simulink model "SIMMODEL"  (R2023b)
settings: Solver=VariableStepAuto  StartTime=0.0  StopTime=1.2  MaxStep=0.2  RelTol=1e-4  EnableMultiTasking=on
libraries: spsThreePhaseFaultLib x12, spsDistributedParametersLineLib x2, spsMutualInductanceLib x2, spsThreePhaseSourceLib x2, spsThreePhaseVIMeasurementLib x1, spspowerguiLib x1
settings Model: Creator=t0197si  LastModifiedBy=takid
settings SolverCC: AlgebraicLoopSolver=TrustRegion  MaxZcPerStep=1
settings DataIOCC: LimitDataPoints=on  MaxDataPoints=10000
settings OptimizationCC: ReuseModelBlockBuffer=off  LifeSpan=inf
settings DebuggingCC: UnconnectedInputMsg=warning  UnconnectedOutputMsg=warning  UnconnectedLineMsg=warning  AllowSymbolicDim=off  SFUnexpectedBacktrackingDiag=warning  SFNoUnconditionalDefaultTransitionDiag=warning  SFExecutionAtInitializationDiag=none  ArithmeticOperatorsInVariantConditions=warning
settings ModelReferenceCC: EnableRefExpFcnMdlSchedulingChecks=on
settings SFSimCC: SimUseLocalCustomCode=off  CustomCodeUndefinedFunction=UseInterfaceOnly
settings RTWCC: RTWUseLocalCustomCode=off  DLArmComputeVersion=19.05
settings CodeAppCC: StateflowObjectComments=on
settings GRTTargetCC: TargetLangStandard=C89/C90 (ANSI)
settings ConfigComp: CovMetricSettings=dw  CovSaveCumulativeToWorkspaceVar=on  CovSaveSingleToWorkspaceVar=on  CovExternalEMLEnable=off  CovSFcnEnable=off
settings SimscapeCC: SimscapeLogType=all  SimscapeLogDataHistory=10000

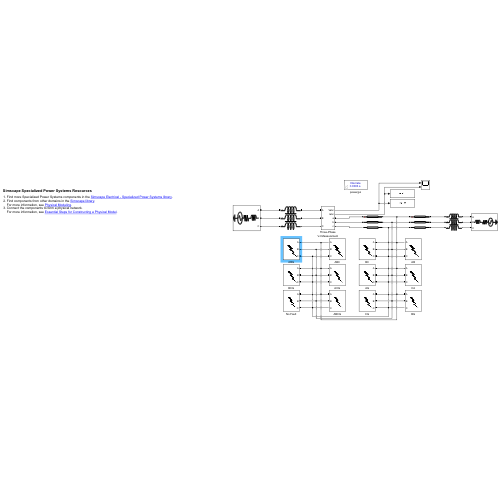
[thumbnail: Simulink's stored preview of the top-level diagram]
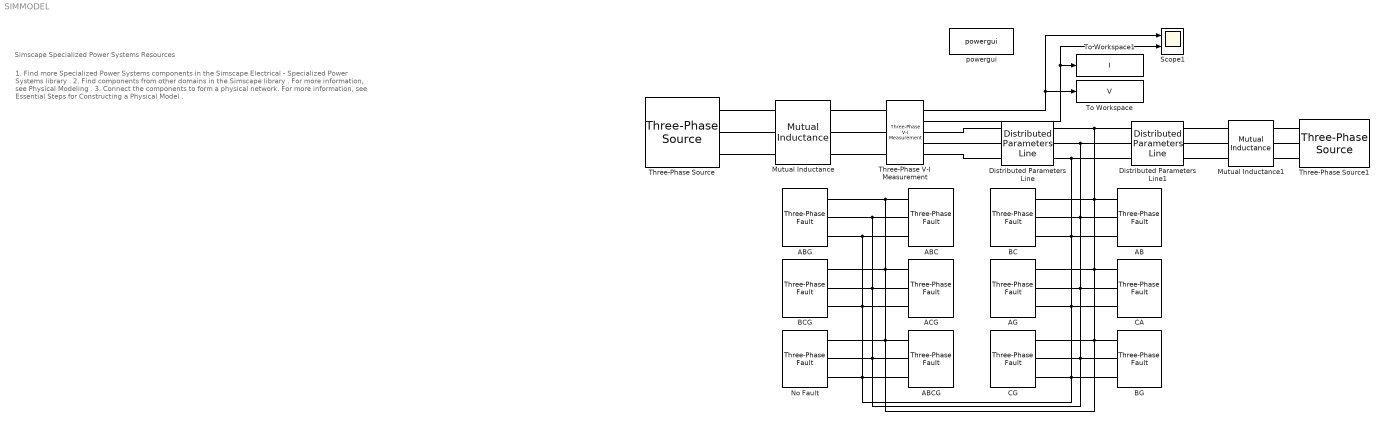
== system SIMMODEL ==
  note: 1. Find more Specialized Power Systems components in the Simscape Electrical - Specialized Power Systems library .
      | 2. Find components from other domains in the Simscape library .
      | For more information, see Physical Modeling .
      | 3. Connect the components to form a physical network.
      | For more information, see Essential Steps for Constructing a Physical Model .
  note: Simscape Specialized Power Systems Resources
  AB : spsThreePhaseFaultLib/Three-Phase Fault  InitialStates=0  FaultA=on  FaultB=on  FaultC=off  GroundFault=off  SwitchTimes="[0.048  0.051]"  External=off  SwitchStatus=NaN  FaultResistance=0.0001  GroundResistance=0.01  SnubberResistance=1e6  SnubberCapacitance=inf  Measurements=Fault voltages and currents
  ABC : spsThreePhaseFaultLib/Three-Phase Fault  InitialStates=0  FaultA=on  FaultB=on  FaultC=on  GroundFault=off  SwitchTimes="[0.648  0.651]"  External=off  SwitchStatus=NaN  FaultResistance=0.0001  GroundResistance=0.01  SnubberResistance=1e6  SnubberCapacitance=inf  Measurements=Fault voltages and currents
  ABCG : spsThreePhaseFaultLib/Three-Phase Fault  InitialStates=0  FaultA=on  FaultB=on  FaultC=on  GroundFault=on  SwitchTimes="[1.05  1.053]"  External=off  SwitchStatus=NaN  FaultResistance=0.0001  GroundResistance=0.01  SnubberResistance=1e6  SnubberCapacitance=inf  Measurements=Fault voltages and currents
  ABG : spsThreePhaseFaultLib/Three-Phase Fault  InitialStates=0  FaultA=on  FaultB=on  FaultC=off  GroundFault=on  SwitchTimes="[0.75  0.753]"  External=off  SwitchStatus=NaN  FaultResistance=0.0001  GroundResistance=0.01  SnubberResistance=1e6  SnubberCapacitance=inf  Measurements=Fault voltages and currents
  ACG : spsThreePhaseFaultLib/Three-Phase Fault  InitialStates=0  FaultA=on  FaultB=off  FaultC=on  GroundFault=on  SwitchTimes="[0.849  0.852]"  External=off  SwitchStatus=NaN  FaultResistance=0.0001  GroundResistance=0.01  SnubberResistance=1e6  SnubberCapacitance=inf  Measurements=Fault voltages and currents
  AG : spsThreePhaseFaultLib/Three-Phase Fault  InitialStates=0  FaultA=on  FaultB=off  FaultC=off  GroundFault=on  SwitchTimes="[0.348  0.351]"  External=off  SwitchStatus=NaN  FaultResistance=0.0001  GroundResistance=0.01  SnubberResistance=1e6  SnubberCapacitance=inf  Measurements=Fault voltages and currents
  BC : spsThreePhaseFaultLib/Three-Phase Fault  InitialStates=0  FaultA=off  FaultB=on  FaultC=on  GroundFault=off  SwitchTimes="[0.150  0.153]"  External=off  SwitchStatus=NaN  FaultResistance=0.0001  GroundResistance=0.01  SnubberResistance=1e6  SnubberCapacitance=inf  Measurements=Fault voltages and currents
  BCG : spsThreePhaseFaultLib/Three-Phase Fault  InitialStates=0  FaultA=off  FaultB=on  FaultC=on  GroundFault=on  SwitchTimes="[0.948  0.951]"  External=off  SwitchStatus=NaN  FaultResistance=0.0001  GroundResistance=0.01  SnubberResistance=1e6  SnubberCapacitance=inf  Measurements=Fault voltages and currents
  BG : spsThreePhaseFaultLib/Three-Phase Fault  InitialStates=0  FaultA=off  FaultB=on  FaultC=off  GroundFault=on  SwitchTimes="[0.45  0.453]"  External=off  SwitchStatus=NaN  FaultResistance=0.0001  GroundResistance=0.01  SnubberResistance=1e6  SnubberCapacitance=inf  Measurements=Fault voltages and currents
  CA : spsThreePhaseFaultLib/Three-Phase Fault  InitialStates=0  FaultA=on  FaultB=off  FaultC=on  GroundFault=off  SwitchTimes="[0.249  0.252]"  External=off  SwitchStatus=NaN  FaultResistance=0.0001  GroundResistance=0.01  SnubberResistance=1e6  SnubberCapacitance=inf  Measurements=Fault voltages and currents
  CG : spsThreePhaseFaultLib/Three-Phase Fault  InitialStates=0  FaultA=off  FaultB=off  FaultC=on  GroundFault=on  SwitchTimes="[0.549  0.552]"  External=off  SwitchStatus=NaN  FaultResistance=0.0001  GroundResistance=0.01  SnubberResistance=1e6  SnubberCapacitance=inf  Measurements=Fault voltages and currents
  Distributed Parameters Line : spsDistributedParametersLineLib/Distributed Parameters Line  Phases=3  Length=100  Frequency=60  Resistance=[0.01273 0.3864]  Inductance="[0.9337e-3  4.1264e-3]"  Capacitance=[12.74e-9 7.751e-9]  x1=[-0.0006 8.38191360726551e-10 366849.409185142 -341970.613327489;-0.0003 9.78318632999942e-10 403099.289377047 -298384.57115405]  x2=[-0.0006 2.49160898759062e-08 369790.162967538 -345071.374185274;-0.0003 2.69712684545462e-08 406371.196257459 -301133.639372877]  x3=[-0.0006 -7.11140025193407e-11 1183.26211569335 -1433.40164787206;-0.0003 -5.12740809092146e-11 1337.47114951323 -1290.70540510875]  x4=[-0.0006 1.02696315275821e-10 1363.36060464342 -1272.22615544696;-0.0003 8.61930580244731e-11 1498.22936173638 -1110.23434847254]  x5=0.000565541566995742  V1=[2.072e-10 5.015e+05 5.015e+05;377 377 377;0.5654 0.9167 -0.6541]  V2=[3.283e-10 5.058e+05 5.058e+05;377 377 377;2.705 0.9161 -0.6547]  I1=[2.823e-12 1859 1859;377 377 377;1.555 0.7863 -0.7845]  I2=[3.303e-12 1865 1865;377 377 377;-0.9037 0.9161 -0.6547]  nHarmo=1  Measurements=None  Decoupling=off  VsMag0=0  VrMag0=0  VsAngle0=0  VrAngle0=0  IsMag0=0  IrMag0=0  IsAngle0=0  IrAngle0=0
      settings: LibrarySourceBlock=sps_lib/Power Grid Elements/Distributed Parameters Line
  Distributed Parameters Line1 : spsDistributedParametersLineLib/Distributed Parameters Line  Phases=3  Length=100  Frequency=60  Resistance=[0.01273 0.3864]  Inductance="[0.9337e-3  4.1264e-3]"  Capacitance=[12.74e-9 7.751e-9]  x1=[-0.0006 2.48987725575321e-08 369790.162967538 -345071.374185274;-0.0003 2.69552313818675e-08 406371.196257459 -301133.639372877]  x2=[-0.0006 1.02377184379559e-09 366849.409185141 -341970.613327489;-0.0003 1.14493289747496e-09 403099.289377047 -298384.57115405]  x3=[-0.0006 1.04415855312855e-10 1363.36060464343 -1272.22615544696;-0.0003 8.82283474754132e-11 1498.22936173639 -1110.23434847254]  x4=[-0.0006 -7.33549795214247e-11 1183.26211569334 -1433.40164787206;-0.0003 -5.35717652018444e-11 1337.47114951323 -1290.70540510875]  x5=0.000565541566995742  V1=[3.185e-10 5.058e+05 5.058e+05;377 377 377;2.745 0.9161 -0.6547]  V2=[1.2e-10 5.015e+05 5.015e+05;377 377 377;-0.4582 0.9167 -0.6541]  I1=[2.458e-12 1865 1865;377 377 377;-1.648 0.9161 -0.6547]  I2=[3.271e-12 1859 1859;377 377 377;1.776 0.7863 -0.7845]  nHarmo=1  Measurements=None  Decoupling=off  VsMag0=0  VrMag0=0  VsAngle0=0  VrAngle0=0  IsMag0=0  IrMag0=0  IsAngle0=0  IrAngle0=0
      settings: LibrarySourceBlock=sps_lib/Power Grid Elements/Distributed Parameters Line
  Mutual Inductance : spsMutualInductanceLib/Mutual Inductance  LConnTagsString=a|b|c  RConnTagsString=A|B|C  TypeOfMutual=Two or three windings with equal mutual terms  NumberOfWindings=3  SelfImpedance1=[1.1 1.1e-03]  SelfImpedance2=[ 1.1 1.1e-03]  ThreeWindings=on  SelfImpedance3=[ 1.1 1.1e-03]  MutualImpedance=[1.0 1.0e-03]  InductanceMatrix="[1.0 0.9  0.9 ;  0.9 1.0  0.9;  0.9 0.9 1.0 ] * 1e-3"  ResistanceMatrix="[1.0 0.9  0.9 ;  0.9 1.0  0.9;  0.9 0.9 1.0 ]"  Measurements=None
      settings: LibrarySourceBlock=sps_lib/Passives/Mutual Inductance
  Mutual Inductance1 : spsMutualInductanceLib/Mutual Inductance  LConnTagsString=a|b|c  RConnTagsString=A|B|C  TypeOfMutual=Two or three windings with equal mutual terms  NumberOfWindings=3  SelfImpedance1=[1.1 1.1e-03]  SelfImpedance2=[ 1.1 1.1e-03]  ThreeWindings=on  SelfImpedance3=[ 1.1 1.1e-03]  MutualImpedance=[1.0 1.0e-03]  InductanceMatrix="[1.0 0.9  0.9 ;  0.9 1.0  0.9;  0.9 0.9 1.0 ] * 1e-3"  ResistanceMatrix="[1.0 0.9  0.9 ;  0.9 1.0  0.9;  0.9 0.9 1.0 ]"  Measurements=None
      settings: LibrarySourceBlock=sps_lib/Passives/Mutual Inductance
  No Fault : spsThreePhaseFaultLib/Three-Phase Fault  InitialStates=0  FaultA=off  FaultB=off  FaultC=off  GroundFault=off  SwitchTimes="[1.15  1.151]"  External=off  SwitchStatus=NaN  FaultResistance=0.0001  GroundResistance=0.01  SnubberResistance=1e6  SnubberCapacitance=inf  Measurements=Fault voltages and currents
  Scope1 : Scope  NumInputPorts=2
  Three-Phase V-I Measurement : spsThreePhaseVIMeasurementLib/Three-Phase V-I Measurement  VoltageMeasurement=phase-to-ground  SetLabelV=off  LabelV=Vabc  Vpu=on  VpuLL=off  CurrentMeasurement=yes  SetLabelI=off  LabelI=Iabc  Ipu=off  Pbase=100e6  Vbase=5e5  OutputType=Complex  PhasorSimulation=off  PSBequivalent=0
  Three-Phase Source : spsThreePhaseSourceLib/Three-Phase Source  InternalConnection=Yg  VoltagePhases=off  Voltage=5e5  PhaseAngle=30  Voltage_phases=[25e3 25e3 25e3]/sqrt(3)  PhaseAngles_phases=[0 -120 +120]  Frequency=60  NonIdealSource=on  SpecifyImpedance=off  Resistance=0.8929  Inductance=16.58e-3  ShortCircuitLevel=100e6  BaseVoltage=25e3  XRratio=7  BusType=swing  Pref=10e3  Qref=0  Prefabc=[10e3, 10e3, 10e3]  Qrefabc=[0, 0, 0]  Qmin=-inf  Qmax=inf
  Three-Phase Source1 : spsThreePhaseSourceLib/Three-Phase Source  InternalConnection=Yg  VoltagePhases=off  Voltage=5e5  PhaseAngle=30  Voltage_phases=[25e3 25e3 25e3]/sqrt(3)  PhaseAngles_phases=[0 -120 +120]  Frequency=60  NonIdealSource=on  SpecifyImpedance=off  Resistance=0.8929  Inductance=16.58e-3  ShortCircuitLevel=100e6  BaseVoltage=25e3  XRratio=7  BusType=swing  Pref=10e3  Qref=0  Prefabc=[10e3, 10e3, 10e3]  Qrefabc=[0, 0, 0]  Qmin=-inf  Qmax=inf
  To Workspace : ToWorkspace  VariableName=V  SampleTime=-1
  To Workspace1 : ToWorkspace  VariableName=I  SampleTime=-1
  powergui : spspowerguiLib/powergui  Priority=1  SimulationMode=Discrete  SampleTime=0.0003  frequency=60  Iterations=50  frequencyindice=60  Pbase=100e6  ErrMax=1e-4  UnitsV=kV  UnitsW=MW  buscounter=0  FunctionMessages=off  echomessages=off  EnableUseOfTLC=off  CurrentSourceSwitches=off  DisableSnubberDevices=off  DisableRonSwitches=off  DisableVfSwitches=off  DisplayEquations=off  AutomaticDiscreteSolvers=off  SolverType=Tustin/Backward Euler (TBE)  Interpol=off  ExternalGateDelay=off  methode=off  Ts=100  x0status=blocks  SPID=on  SwTol=0  HookPort=off  NonlinearTolerance=0  nMaxIteration=15  ContinueOnMaxIteration=off  RestoreLinks=warning  ResistiveCurrentMeasurement=off  Frange=[0:2:500]  Ylog=off  Xlog=on  ShowGrid=off  save=off  variable=ZData  structure=0  ZoomFFT=off  StartTime=0.0  cycles=1  DisplayStyle=1  fundamental=60  FreqAxis=off  MaxFrequency=1000  frequencyindicesteady=1  RmsSteady=1  display=off
  wires:
  Three-Phase V-I Measurement/1 -> Scope1/1, To Workspace/1
  Three-Phase V-I Measurement/2 -> Scope1/2, To Workspace1/1
  connections:
  Three-Phase Source/RConn1 -- Mutual Inductance/LConn1
  Three-Phase Source/RConn2 -- Mutual Inductance/LConn2
  Three-Phase Source/RConn3 -- Mutual Inductance/LConn3
  Mutual Inductance/RConn1 -- Three-Phase V-I Measurement/LConn1
  Mutual Inductance/RConn2 -- Three-Phase V-I Measurement/LConn2
  Mutual Inductance/RConn3 -- Three-Phase V-I Measurement/LConn3
  Three-Phase V-I Measurement/RConn1 -- Distributed Parameters Line/LConn1
  Three-Phase V-I Measurement/RConn2 -- Distributed Parameters Line/LConn2
  Three-Phase V-I Measurement/RConn3 -- Distributed Parameters Line/LConn3
  Mutual Inductance1/LConn1 -- Distributed Parameters Line1/RConn1
  Mutual Inductance1/LConn2 -- Distributed Parameters Line1/RConn2
  Mutual Inductance1/LConn3 -- Distributed Parameters Line1/RConn3
  Mutual Inductance1/RConn1 -- Three-Phase Source1/RConn1
  Mutual Inductance1/RConn2 -- Three-Phase Source1/RConn2
  Mutual Inductance1/RConn3 -- Three-Phase Source1/RConn3
  Distributed Parameters Line1/LConn1 -- AB/LConn1 -- BC/LConn1 -- AG/LConn1 -- CA/LConn1 -- ABCG/LConn1 -- No Fault/LConn1 -- ACG/LConn1 -- BCG/LConn1 -- ABC/LConn1 -- ABG/LConn1 -- CG/LConn1 -- BG/LConn1 -- Distributed Parameters Line/RConn1
  Distributed Parameters Line1/LConn2 -- ABCG/LConn2 -- ABG/LConn2 -- ABC/LConn2 -- BCG/LConn2 -- ACG/LConn2 -- No Fault/LConn2 -- CG/LConn2 -- BG/LConn2 -- AG/LConn2 -- CA/LConn2 -- BC/LConn2 -- AB/LConn2 -- Distributed Parameters Line/RConn2
  Distributed Parameters Line1/LConn3 -- CG/LConn3 -- ABG/LConn3 -- ABC/LConn3 -- BCG/LConn3 -- ACG/LConn3 -- No Fault/LConn3 -- ABCG/LConn3 -- BG/LConn3 -- AG/LConn3 -- CA/LConn3 -- BC/LConn3 -- AB/LConn3 -- Distributed Parameters Line/RConn3
